simulink model "UnicycleWithSensor2019b"  (R2021a)
settings: Solver=VariableStepAuto  StartTime=0.0  StopTime=10.0  RelTol=1e-3
values from neighbouring files (symbols this model uses):
  P = 10    [go2goalWithSensor.m]
  thetainit = 0    [go2goalWithSensor.m]
  v = 1    [go2goalWithSensor.m]
  xg = gPos(2)    [go2goalWithSensor.m]
  xinit = sPos(2)    [go2goalWithSensor.m]
  yg = gPos(1)    [go2goalWithSensor.m]
  yinit = sPos(1)    [go2goalWithSensor.m]
  Z = ones(SizeX, SizeY)*255    [CreateMaze.m]
libraries: pid_lib x1
settings Model: Creator=npn01  LastModifiedBy=vp96
settings SolverCC: AlgebraicLoopSolver=TrustRegion
settings DebuggingCC: SFMachineParentedDataDiag=warning  ArithmeticOperatorsInVariantConditions=warning
settings SFSimCC: CustomCodeUndefinedFunction=UseInterfaceOnly

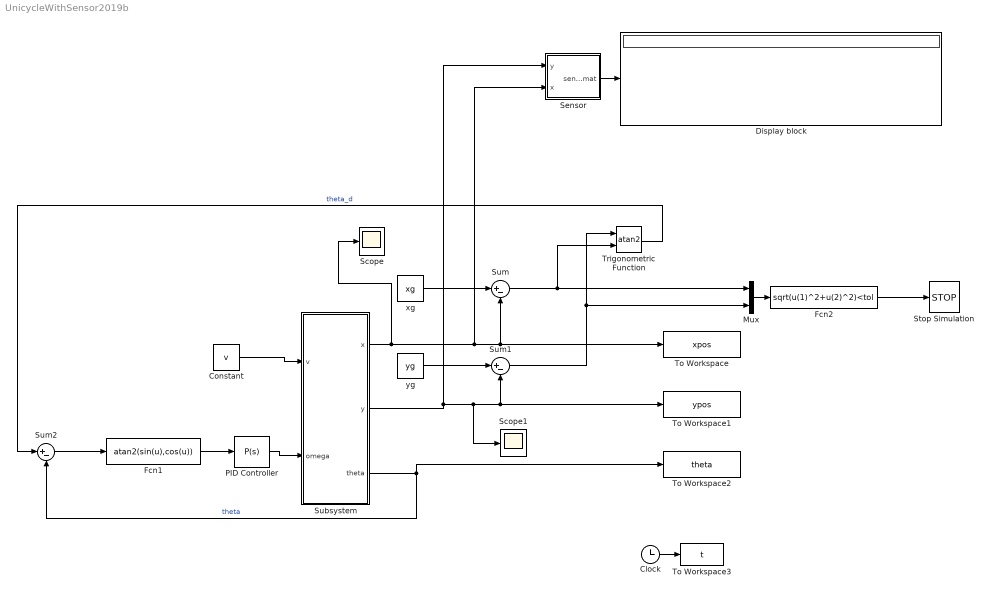
== system UnicycleWithSensor2019b ==
  Clock : Clock
  Constant : Constant  Value=v
  Display block : Display
  Fcn1 : Fcn  Expr=atan2(sin(u),cos(u))
  Fcn2 : Fcn  Expr=sqrt(u(1)^2+u(2)^2)<tol
  Mux : Mux  Inputs=2
  PID Controller : pid_lib/PID Controller  Controller=P  Form=Parallel  TimeDomain=Continuous-time  UseExternalTs=off  SampleTime=-1  IntegratorMethod=Forward Euler  FilterMethod=Forward Euler  ControllerParametersSource=internal  P=P  I=0  D=0  UseFilter=on  N=100  TunerSelectOption=Transfer Function Based (PID Tuner App)  InitialConditionSource=internal  InitialConditionForIntegrator=0  InitialConditionForFilter=0  DifferentiatorICPrevScaledInput=0  ExternalReset=none  TrackingMode=off  Kt=1  LimitOutput=off  SatLimitsSource=internal  UpperSaturationLimit=inf  LowerSaturationLimit=-inf  LinearizeAsGain=on  AntiWindupMode=none  Kb=1  POutMin=[]  POutMax=[]  IOutMin=[]  IOutMax=[]  DOutMin=[]  DOutMax=[]  NOutMin=[]  NOutMax=[]  SumOutMin=[]  SumOutMax=[]  SaturationOutMin=[]  SaturationOutMax=[]  PParamMin=[]  PParamMax=[]  IParamMin=[]  IParamMax=[]  DParamMin=[]  DParamMax=[]  NParamMin=[]  NParamMax=[]  KbParamMin=[]  KbParamMax=[]  KtParamMin=[]  KtParamMax=[]  KbOutMin=[]  KbOutMax=[]  KtOutMin=[]  KtOutMax=[]  IntegratorOutMin=[]  IntegratorOutMax=[]  FilterOutMin=[]  FilterOutMax=[]  SumI1OutMin=[]  SumI1OutMax=[]  SumI2OutMin=[]  SumI2OutMax=[]  SumI3OutMin=[]  SumI3OutMax=[]  SumI4OutMin=[]  SumI4OutMax=[]  SumDOutMin=[]  SumDOutMax=[]  DifferentiatorOutMin=[]  DifferentiatorOutMax=[]  FilterDiffOutCoefMin=[]  FilterDiffOutCoefMax=[]  ReciprocalOutMin=[]  ReciprocalOutMax=[]  SumDenOutMin=[]  SumDenOutMax=[]  SumNumOutMin=[]  SumNumOutMax=[]  DivideOutMin=[]  DivideOutMax=[]  UdiffTsProdOutMin=[]  UdiffTsProdOutMax=[]  NTsProdOutMin=[]  NTsProdOutMax=[]  UintegralTsProdOutMin=[]  UintegralTsProdOutMax=[]  UngainTsProdOutMin=[]  UngainTsProdOutMax=[]  IntegratorContinuousStateAttributes=''  IntegratorStateMustResolveToSignalObject=off  IntegratorRTWStateStorageClass=Auto  FilterContinuousStateAttributes=''  FilterStateMustResolveToSignalObject=off  FilterRTWStateStorageClass=Auto  ParallelPVariant=InternalParameters  IdealPVariant=Disabled  IVariant=Disabled  DVariant=Disabled  IntegratorVariant=Disabled  SatVariant=Disabled  AWVariant=Disabled  PCopyVariant=Disabled  TRVariant=Disabled  FdbkBlocksVariant=Forward  IdealPFdbkVariant=Disabled  SatFdbkVariant=Disabled  DerivativeFilterVariant=Disabled  NVariant=Disabled  NCopyVariant=Disabled_SignalSpec  FilterICVariant=Disabled  IntegratorICVariant=Disabled  ExternalResetVariant=Disabled  TRSumVariant=Passthrough  SumFdbkVariant=Disabled  SumVariant=Passthrough_P  TsampFilterVariant=InternalTs  TsampNgainVariant=Passthrough  TsampIntegralVariant=Disabled_SignalSpec  ExternalSaturationOutDataTypeStr=Inherit: Same as second input
  Scope : Scope
  Scope1 : Scope
  Sensor : Subsystem
  Stop Simulation : Stop
  Subsystem : Subsystem  mask{x0=xinit, y0=yinit, theta0=thetainit}
      mask DialogControl Control4 Prompt: Enter x initial position
      mask DialogControl Control2 Prompt: Enter y initial position
      mask DialogControl Control3 Prompt: Enter initial theta angle
      mask DialogControl Control6 Prompt: Any text you want
  Sum : Sum  Inputs=|+-
  Sum1 : Sum  Inputs=|+-
  Sum2 : Sum  Inputs=|+-
  To Workspace : ToWorkspace  VariableName=xpos  SampleTime=-1
  To Workspace1 : ToWorkspace  VariableName=ypos  SampleTime=-1
  To Workspace2 : ToWorkspace  VariableName=theta  SampleTime=-1
  To Workspace3 : ToWorkspace  VariableName=t  SampleTime=-1
      settings: Save2DSignal=2-D array (concatenate along first dimension)
  Trigonometric Function : Trigonometry  Operator=atan2
  xg : Constant  Value=xg
  yg : Constant  Value=yg
  wires:
  Constant/1 -> Subsystem/1(v)
  xg/1 -> Sum/1
  Subsystem/1(x) -> Scope/1, Sensor/2(x), To Workspace/1, Sum/2
  yg/1 -> Sum1/1
  Subsystem/2(y) -> Sensor/1(y), Scope1/1, Sum1/2, To Workspace1/1
  Sum/1 -> Trigonometric Function/2, Mux/1
  Subsystem/3(theta) -> To Workspace2/1, Sum2/2  "theta"
  Trigonometric Function/1 -> Sum2/1  "theta_d"
  PID Controller/1 -> Subsystem/2(omega)
  Sum2/1 -> Fcn1/1
  Fcn1/1 -> PID Controller/1
  Clock/1 -> To Workspace3/1
  Mux/1 -> Fcn2/1
  Sum1/1 -> Trigonometric Function/1, Mux/2
  Fcn2/1 -> Stop Simulation/1
  Sensor/1(sensor_mat) -> Display block/1

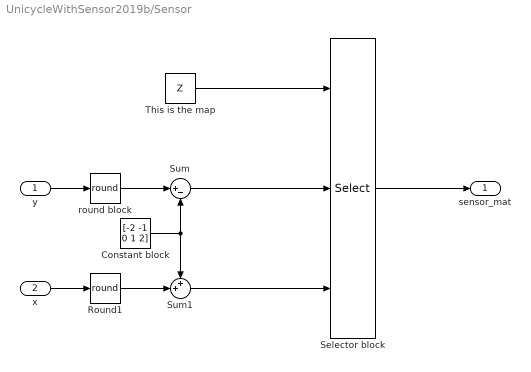
== system UnicycleWithSensor2019b/Sensor ==
  y : Inport
  x : Inport  Port=2
  Constant block : Constant  Value=[-2 -1 0 1 2]
  Round1 : Rounding  Operator=round
  Selector block : Selector  NumberOfDimensions=2  InputPortWidth=3  IndexOptions=Index vector (port),Index vector (port)  Indices=[1 3],1  OutputSizes=1,1
  Sum : Sum  Inputs=|+-  OutDataTypeStr=int32  RndMeth=Round
  Sum1 : Sum  Inputs=++|  OutDataTypeStr=int32  RndMeth=Round
  This is the map : Constant  Value=Z  VectorParams1D=off
  round block : Rounding  Operator=round
  sensor_mat : Outport
  wires:
  This is the map/1 -> Selector block/1
  Constant block/1 -> Sum1/1, Sum/2
  Sum/1 -> Selector block/2
  Sum1/1 -> Selector block/3
  Selector block/1 -> sensor_mat/1
  y/1 -> round block/1
  round block/1 -> Sum/1
  x/1 -> Round1/1
  Round1/1 -> Sum1/2

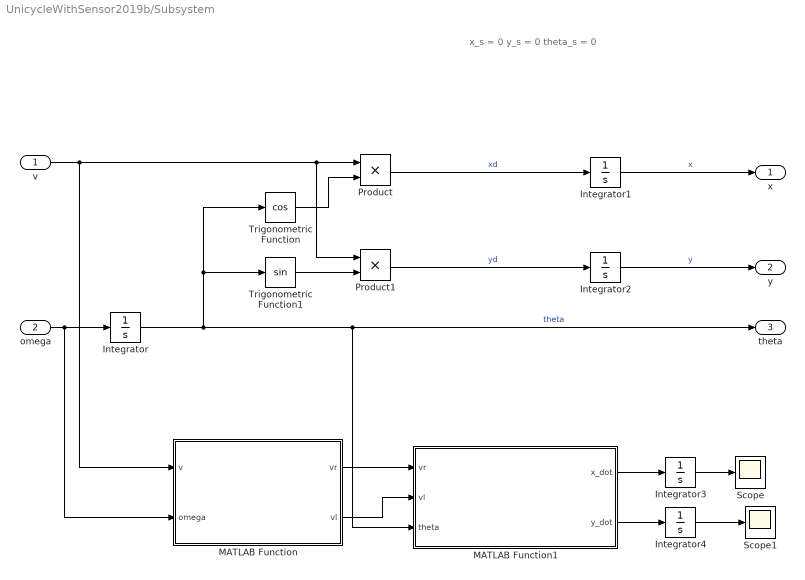
== system UnicycleWithSensor2019b/Subsystem ==
  note: x_s = 0
      | y_s = 0
      | theta_s = 0
  v : Inport
  omega : Inport  Port=2
  Integrator : Integrator  InitialCondition=theta0
  Integrator1 : Integrator  InitialCondition=x0
  Integrator2 : Integrator  InitialCondition=y0
  Integrator3 : Integrator
  Integrator4 : Integrator
  MATLAB Function : MATLAB Function  TreatAsAtomicUnit=on
  MATLAB Function1 : MATLAB Function  TreatAsAtomicUnit=on
  Product : Product
  Product1 : Product
  Scope : Scope
  Scope1 : Scope
  Trigonometric Function : Trigonometry  Operator=cos
  Trigonometric Function1 : Trigonometry
  x : Outport
  y : Outport  Port=2
  theta : Outport  Port=3
  wires:
  Product1/1 -> Integrator2/1  "yd"
  Integrator2/1 -> y/1  "y"
  v/1 -> MATLAB Function/1(v), Product1/1, Product/1
  Integrator/1 -> MATLAB Function1/3(theta), theta/1, Trigonometric Function1/1, Trigonometric Function/1  "theta"
  Product/1 -> Integrator1/1  "xd"
  omega/1 -> MATLAB Function/2(omega), Integrator/1
  Trigonometric Function/1 -> Product/2
  Integrator1/1 -> x/1  "x"
  Trigonometric Function1/1 -> Product1/2
  MATLAB Function/1(vr) -> MATLAB Function1/1(vr)
  MATLAB Function/2(vl) -> MATLAB Function1/2(vl)
  MATLAB Function1/1(x_dot) -> Integrator3/1
  MATLAB Function1/2(y_dot) -> Integrator4/1
  Integrator3/1 -> Scope/1
  Integrator4/1 -> Scope1/1

== matlab function UnicycleWithSensor2019b/Subsystem/MATLAB Function1 ==
  data: vr input; x_dot output; vl input; theta input; y_dot output
function [x_dot,y_dot] = velocity_from_differential(vr,vl,theta)
    r = 0.1;
    l = 0.5;
    x_dot = (r/2)*(vr+vl)*cos(theta);
    y_dot = (r/2)*(vr+vl)*sin(theta);

== matlab function UnicycleWithSensor2019b/Subsystem/MATLAB Function ==
  data: v input; vr output; omega input; vl output
function [vr,vl] = differential_from_theta(v,omega)
    r = 0.1;
    l = 0.5;
    vr = (2*v+omega*l)/(2*r);
    vl = (2*v-omega*l)/(2*r);
